simulink model "On_Board_Computer"  (R2024a)
settings: Solver=FixedStepAuto  StartTime=0.0  StopTime=10  FixedStep=sampleTime  RelTol=1e-3
values from neighbouring files (symbols this model uses):
  gains =     [workspace.mat]
settings Model: Creator=matteocolussi  LastModifiedBy=matteocolussi
settings DataIOCC: SaveOutput=off  SaveTime=off
settings ModelReferenceCC: UseModelRefSolver=on

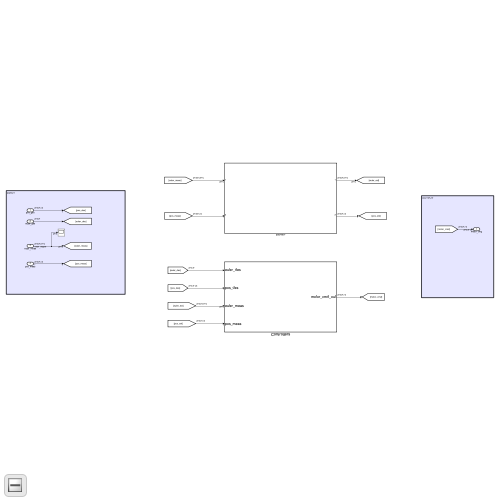
[thumbnail: Simulink's stored preview of the top-level diagram]
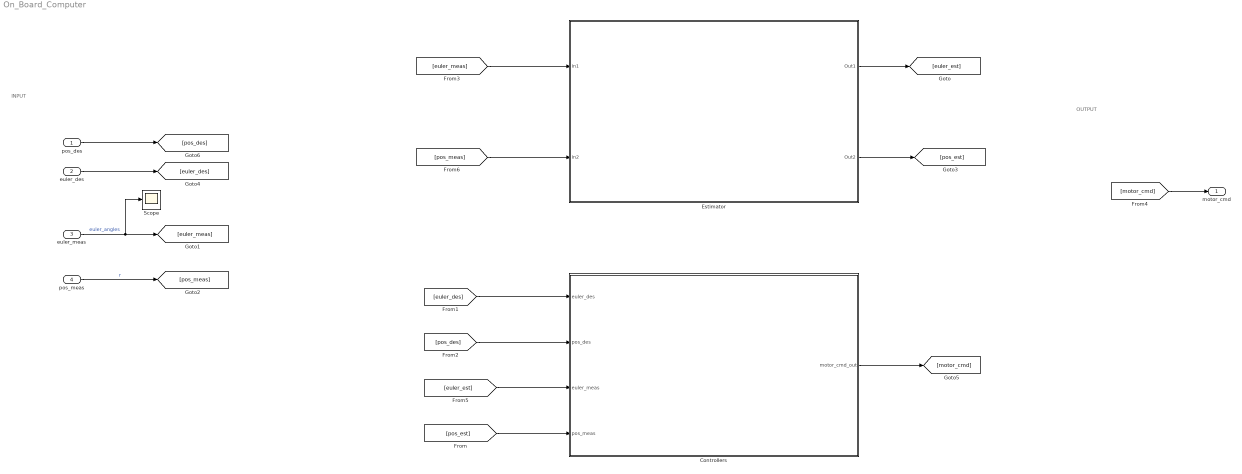
== system On_Board_Computer ==
  note: INPUT
  note: OUTPUT
  pos_des : Inport  OutDataTypeStr=double  PortDimensions=3
  euler_des : Inport  Port=2  OutDataTypeStr=double  PortDimensions=1
  euler_meas : Inport  Port=3  OutDataTypeStr=double  PortDimensions=[3 1]  SampleTime=0
  pos_meas : Inport  Port=4  OutDataTypeStr=double  PortDimensions=3  SampleTime=0
  Controllers : Subsystem
  Estimator : Subsystem
  Scope : Scope
  motor_cmd : Outport  OutDataTypeStr=double  PortDimensions=4  SampleTime=0
  wires:
  [euler_des] -> Controllers/1(euler_des)
  pos_des/1 -> [pos_des]
  pos_meas/1 -> [pos_meas]  "r"
  [pos_meas] -> Estimator/2(In2)
  [euler_meas] -> Estimator/1(In1)
  [pos_est] -> Controllers/4(pos_meas)
  euler_meas/1 -> Scope/1, [euler_meas]  "euler_angles"
  [motor_cmd] -> motor_cmd/1
  euler_des/1 -> [euler_des]
  [pos_des] -> Controllers/2(pos_des)
  Estimator/2(Out2) -> [pos_est]
  Estimator/1(Out1) -> [euler_est]
  [euler_est] -> Controllers/3(euler_meas)
  Controllers/1(motor_cmd_out) -> [motor_cmd]

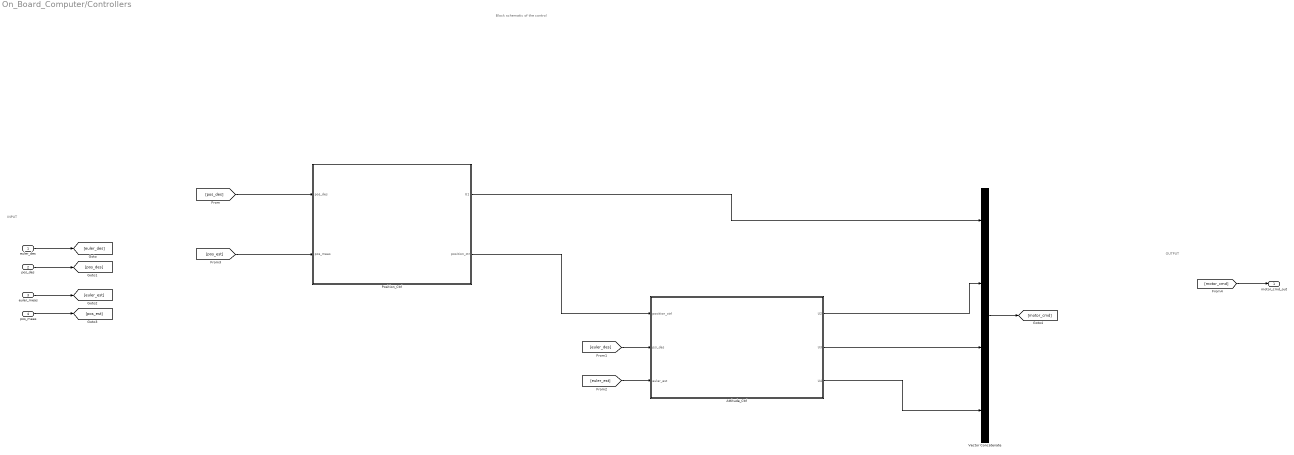
== system On_Board_Computer/Controllers ==
  note: INPUT
  note: OUTPUT
  note: Block schematic of the control
  euler_des : Inport
  pos_des : Inport  Port=2
  euler_meas : Inport  Port=3
  pos_meas : Inport  Port=4
  Attitude_Ctrl : Subsystem
  Position_Ctrl : Subsystem
  Vector Concatenate : Concatenate  NumInputs=4
  motor_cmd_out : Outport
  wires:
  [euler_des] -> Attitude_Ctrl/2(psi_des)
  Vector Concatenate/1 -> [motor_cmd]
  Attitude_Ctrl/3(U4) -> Vector Concatenate/4
  Attitude_Ctrl/2(U3) -> Vector Concatenate/3
  Attitude_Ctrl/1(U2) -> Vector Concatenate/2
  Position_Ctrl/1(U1) -> Vector Concatenate/1
  Position_Ctrl/2(position_ctrl) -> Attitude_Ctrl/1(position_ctrl)
  [pos_des] -> Position_Ctrl/1(pos_des)
  [pos_est] -> Position_Ctrl/2(pos_meas)
  [motor_cmd] -> motor_cmd_out/1
  [euler_est] -> Attitude_Ctrl/3(euler_est)
  euler_meas/1 -> [euler_est]
  pos_meas/1 -> [pos_est]
  pos_des/1 -> [pos_des]
  euler_des/1 -> [euler_des]

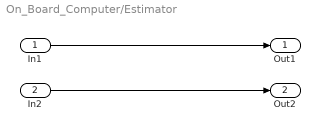
== system On_Board_Computer/Estimator ==
  In1 : Inport
  In2 : Inport  Port=2
  Out1 : Outport
  Out2 : Outport  Port=2
  wires:
  In2/1 -> Out2/1
  In1/1 -> Out1/1

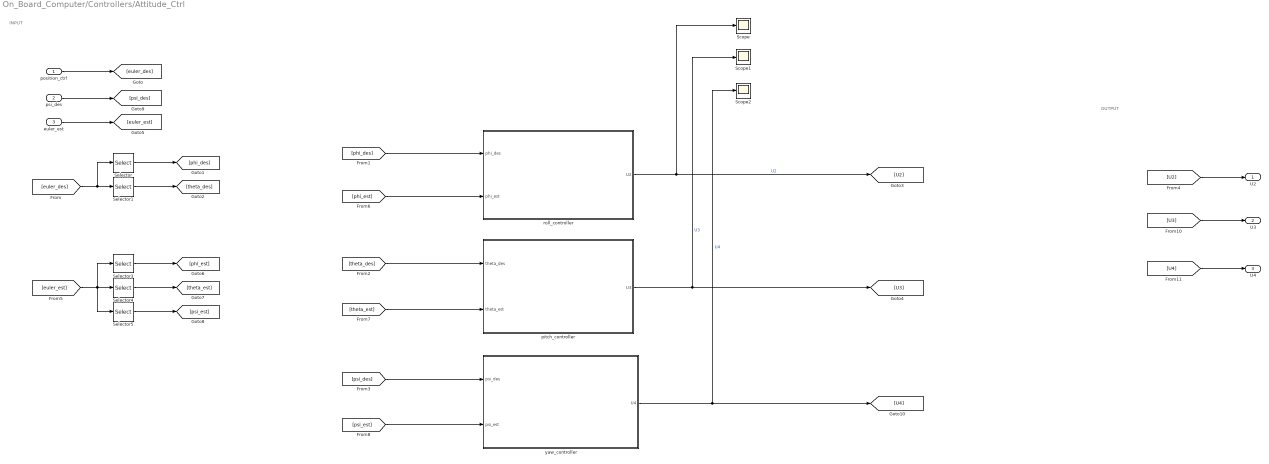
== system On_Board_Computer/Controllers/Attitude_Ctrl ==
  note: INPUT
  note: OUTPUT
  position_ctrl : Inport
  psi_des : Inport  Port=2
  euler_est : Inport  Port=3
  Scope : Scope
  Scope1 : Scope
  Scope2 : Scope
  Selector : Selector  InputPortWidth=2  IndexOptions=Index vector (dialog)  Indices=1  OutputSizes=1
  Selector1 : Selector  InputPortWidth=2  IndexOptions=Index vector (dialog)  Indices=2  OutputSizes=1
  Selector3 : Selector  InputPortWidth=3  IndexOptions=Index vector (dialog)  Indices=1  OutputSizes=1
  Selector4 : Selector  InputPortWidth=3  IndexOptions=Index vector (dialog)  Indices=2  OutputSizes=1
  Selector5 : Selector  InputPortWidth=3  IndexOptions=Index vector (dialog)  Indices=3  OutputSizes=1
  pitch_controller : Subsystem
  roll_controller : Subsystem
  yaw_controller : Subsystem
  U2 : Outport
  U3 : Outport  Port=2
  U4 : Outport  Port=3
  wires:
  psi_des/1 -> [psi_des]
  [U4] -> U4/1
  [U3] -> U3/1
  [U2] -> U2/1
  Selector3/1 -> [phi_est]
  Selector5/1 -> [psi_est]
  Selector4/1 -> [theta_est]
  [euler_est] -> Selector3/1, Selector4/1, Selector5/1
  Selector1/1 -> [theta_des]
  [euler_des] -> Selector/1, Selector1/1
  Selector/1 -> [phi_des]
  [psi_est] -> yaw_controller/2(psi_est)
  [theta_est] -> pitch_controller/2(theta_est)
  [phi_est] -> roll_controller/2(phi_est)
  euler_est/1 -> [euler_est]
  yaw_controller/1(U4) -> Scope2/1, [U4]  "U4"
  pitch_controller/1(U3) -> Scope1/1, [U3]  "U3"
  roll_controller/1(U2) -> Scope/1, [U2]  "U2"
  [psi_des] -> yaw_controller/1(psi_des)
  [theta_des] -> pitch_controller/1(theta_des)
  [phi_des] -> roll_controller/1(phi_des)
  position_ctrl/1 -> [euler_des]

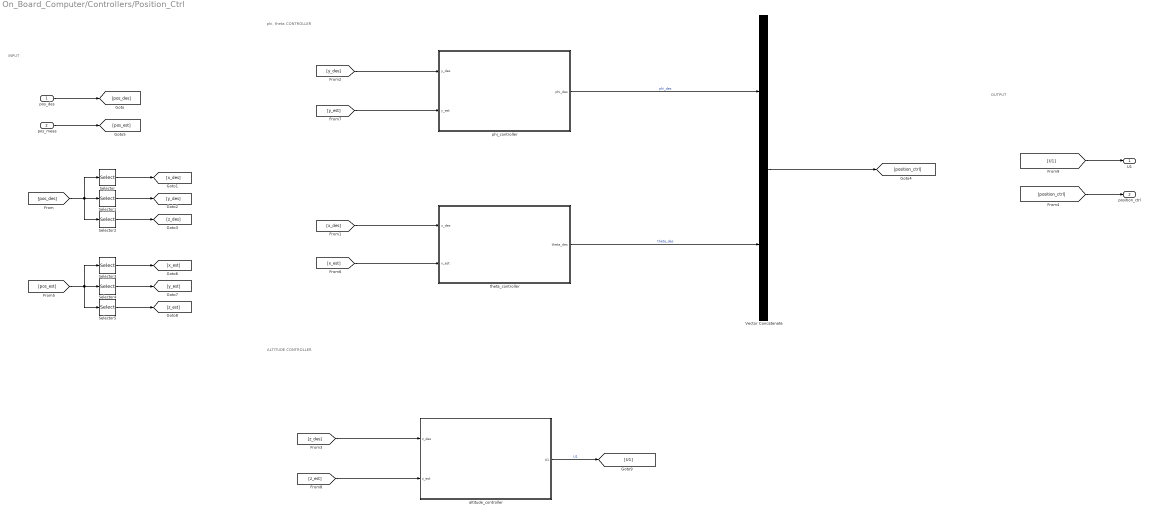
== system On_Board_Computer/Controllers/Position_Ctrl ==
  note: OUTPUT
  note: INPUT
  note: phi, theta CONTROLLER
  note: ALTITUDE CONTROLLER
  pos_des : Inport
  pos_meas : Inport  Port=2
  Selector : Selector  InputPortWidth=3  IndexOptions=Index vector (dialog)  Indices=1  OutputSizes=1
  Selector1 : Selector  InputPortWidth=3  IndexOptions=Index vector (dialog)  Indices=2  OutputSizes=1
  Selector2 : Selector  InputPortWidth=3  IndexOptions=Index vector (dialog)  Indices=3  OutputSizes=1
  Selector3 : Selector  InputPortWidth=3  IndexOptions=Index vector (dialog)  Indices=1  OutputSizes=1
  Selector4 : Selector  InputPortWidth=3  IndexOptions=Index vector (dialog)  Indices=2  OutputSizes=1
  Selector5 : Selector  InputPortWidth=3  IndexOptions=Index vector (dialog)  Indices=3  OutputSizes=1
  Vector Concatenate : Concatenate
  altitude_controller : Subsystem
  phi_controller : Subsystem
  theta_controller : Subsystem
  U1 : Outport
  position_ctrl : Outport  Port=2
  wires:
  phi_controller/1(phi_des) -> Vector Concatenate/1  "phi_des"
  [U1] -> U1/1
  altitude_controller/1(U1) -> [U1]  "U1"
  [z_des] -> altitude_controller/1(z_des)
  [z_est] -> altitude_controller/2(z_est)
  theta_controller/1(theta_des) -> Vector Concatenate/2  "theta_des"
  Vector Concatenate/1 -> [position_ctrl]
  [position_ctrl] -> position_ctrl/1
  [x_est] -> theta_controller/2(x_est)
  [y_des] -> phi_controller/1(y_des)
  [x_des] -> theta_controller/1(x_des)
  [y_est] -> phi_controller/2(y_est)
  Selector2/1 -> [z_des]
  Selector1/1 -> [y_des]
  pos_des/1 -> [pos_des]
  Selector/1 -> [x_des]
  [pos_des] -> Selector/1, Selector1/1, Selector2/1
  Selector5/1 -> [z_est]
  pos_meas/1 -> [pos_est]
  [pos_est] -> Selector3/1, Selector4/1, Selector5/1
  Selector4/1 -> [y_est]
  Selector3/1 -> [x_est]

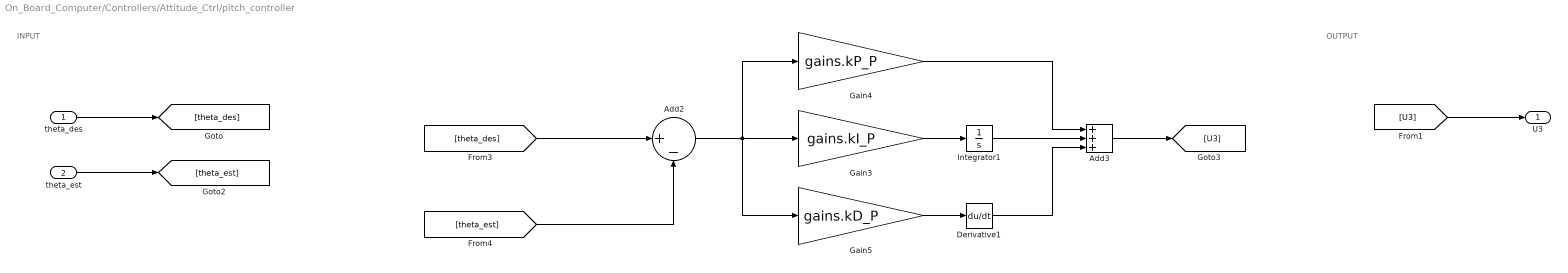
== system On_Board_Computer/Controllers/Attitude_Ctrl/pitch_controller ==
  note: INPUT
  note: OUTPUT
  theta_des : Inport
  theta_est : Inport  Port=2
  Add2 : Sum  Inputs=|+-
  Add3 : Sum  Inputs=+++
  Derivative1 : Derivative
  Gain3 : Gain  Gain=gains.kI_P
  Gain4 : Gain  Gain=gains.kP_P
  Gain5 : Gain  Gain=gains.kD_P
  Integrator1 : Integrator
  U3 : Outport
  wires:
  Gain3/1 -> Integrator1/1
  Gain5/1 -> Derivative1/1
  Add2/1 -> Gain3/1, Gain4/1, Gain5/1
  Integrator1/1 -> Add3/2
  [theta_est] -> Add2/2
  Derivative1/1 -> Add3/3
  Add3/1 -> [U3]
  Gain4/1 -> Add3/1
  [theta_des] -> Add2/1
  theta_est/1 -> [theta_est]
  theta_des/1 -> [theta_des]
  [U3] -> U3/1

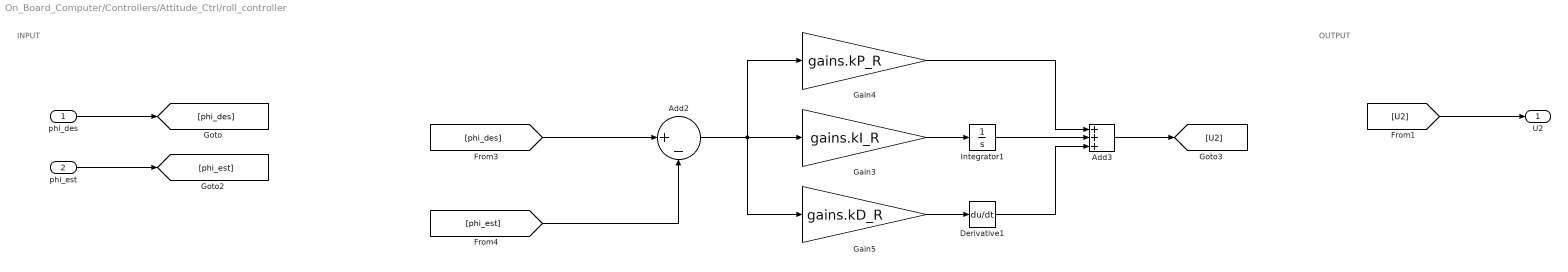
== system On_Board_Computer/Controllers/Attitude_Ctrl/roll_controller ==
  note: INPUT
  note: OUTPUT
  phi_des : Inport
  phi_est : Inport  Port=2
  Add2 : Sum  Inputs=|+-
  Add3 : Sum  Inputs=+++
  Derivative1 : Derivative
  Gain3 : Gain  Gain=gains.kI_R
  Gain4 : Gain  Gain=gains.kP_R
  Gain5 : Gain  Gain=gains.kD_R
  Integrator1 : Integrator
  U2 : Outport
  wires:
  Gain3/1 -> Integrator1/1
  Gain5/1 -> Derivative1/1
  Add2/1 -> Gain3/1, Gain4/1, Gain5/1
  Integrator1/1 -> Add3/2
  [phi_est] -> Add2/2
  Derivative1/1 -> Add3/3
  Add3/1 -> [U2]
  Gain4/1 -> Add3/1
  [phi_des] -> Add2/1
  phi_est/1 -> [phi_est]
  [U2] -> U2/1
  phi_des/1 -> [phi_des]

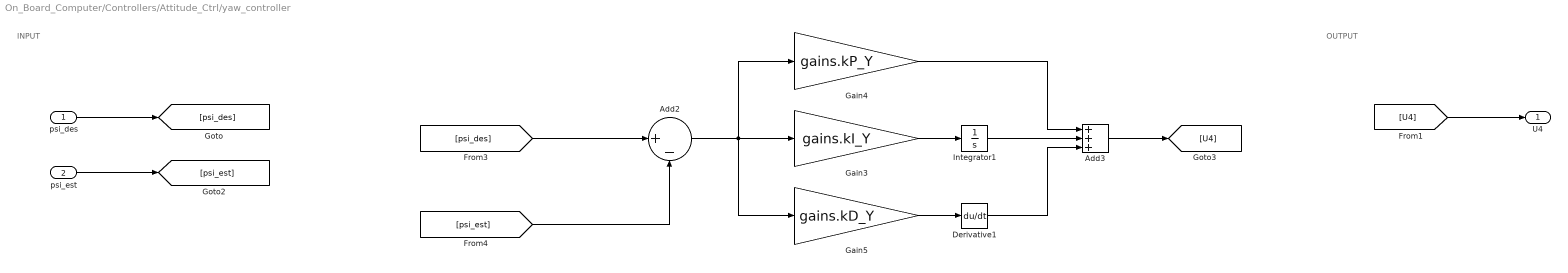
== system On_Board_Computer/Controllers/Attitude_Ctrl/yaw_controller ==
  note: INPUT
  note: OUTPUT
  psi_des : Inport
  psi_est : Inport  Port=2
  Add2 : Sum  Inputs=|+-
  Add3 : Sum  Inputs=+++
  Derivative1 : Derivative
  Gain3 : Gain  Gain=gains.kI_Y
  Gain4 : Gain  Gain=gains.kP_Y
  Gain5 : Gain  Gain=gains.kD_Y
  Integrator1 : Integrator
  U4 : Outport
  wires:
  Gain3/1 -> Integrator1/1
  Gain5/1 -> Derivative1/1
  Add2/1 -> Gain3/1, Gain4/1, Gain5/1
  Integrator1/1 -> Add3/2
  [psi_est] -> Add2/2
  Derivative1/1 -> Add3/3
  Add3/1 -> [U4]
  Gain4/1 -> Add3/1
  [psi_des] -> Add2/1
  psi_est/1 -> [psi_est]
  psi_des/1 -> [psi_des]
  [U4] -> U4/1

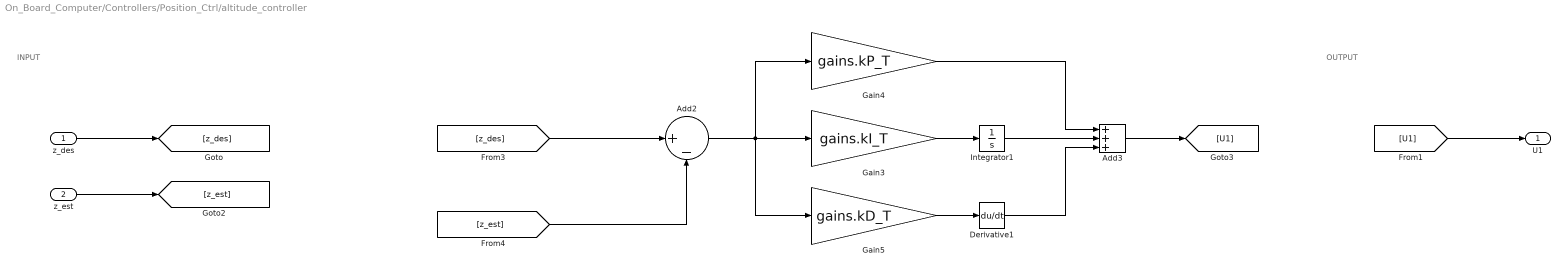
== system On_Board_Computer/Controllers/Position_Ctrl/altitude_controller ==
  note: INPUT
  note: OUTPUT
  z_des : Inport
  z_est : Inport  Port=2
  Add2 : Sum  Inputs=|+-
  Add3 : Sum  Inputs=+++
  Derivative1 : Derivative
  Gain3 : Gain  Gain=gains.kI_T
  Gain4 : Gain  Gain=gains.kP_T
  Gain5 : Gain  Gain=gains.kD_T
  Integrator1 : Integrator
  U1 : Outport
  wires:
  Gain3/1 -> Integrator1/1
  Gain5/1 -> Derivative1/1
  Add2/1 -> Gain3/1, Gain4/1, Gain5/1
  Integrator1/1 -> Add3/2
  [z_est] -> Add2/2
  Derivative1/1 -> Add3/3
  Add3/1 -> [U1]
  Gain4/1 -> Add3/1
  [z_des] -> Add2/1
  z_est/1 -> [z_est]
  z_des/1 -> [z_des]
  [U1] -> U1/1

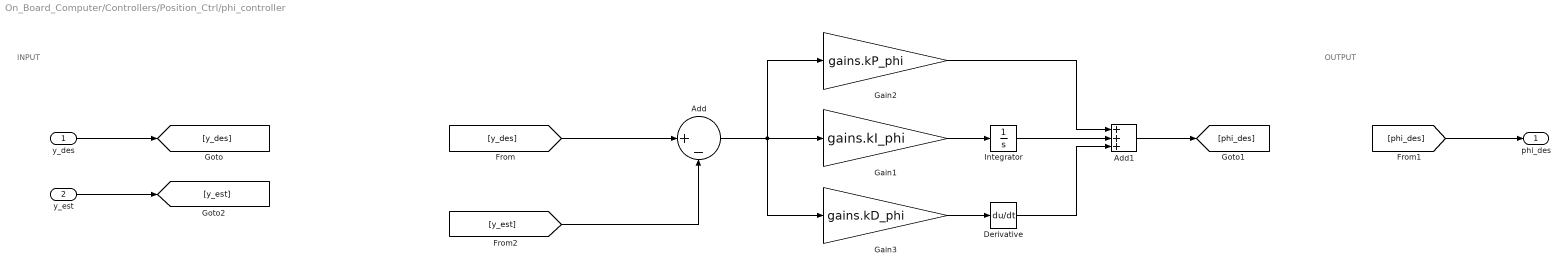
== system On_Board_Computer/Controllers/Position_Ctrl/phi_controller ==
  note: INPUT
  note: OUTPUT
  y_des : Inport
  y_est : Inport  Port=2
  Add : Sum  Inputs=|+-
  Add1 : Sum  Inputs=+++
  Derivative : Derivative
  Gain1 : Gain  Gain=gains.kI_phi
  Gain2 : Gain  Gain=gains.kP_phi
  Gain3 : Gain  Gain=gains.kD_phi
  Integrator : Integrator
  phi_des : Outport
  wires:
  Gain3/1 -> Derivative/1
  Add1/1 -> [phi_des]
  Derivative/1 -> Add1/3
  Gain2/1 -> Add1/1
  Add/1 -> Gain1/1, Gain2/1, Gain3/1
  Gain1/1 -> Integrator/1
  Integrator/1 -> Add1/2
  [y_est] -> Add/2
  y_est/1 -> [y_est]
  y_des/1 -> [y_des]
  [y_des] -> Add/1
  [phi_des] -> phi_des/1

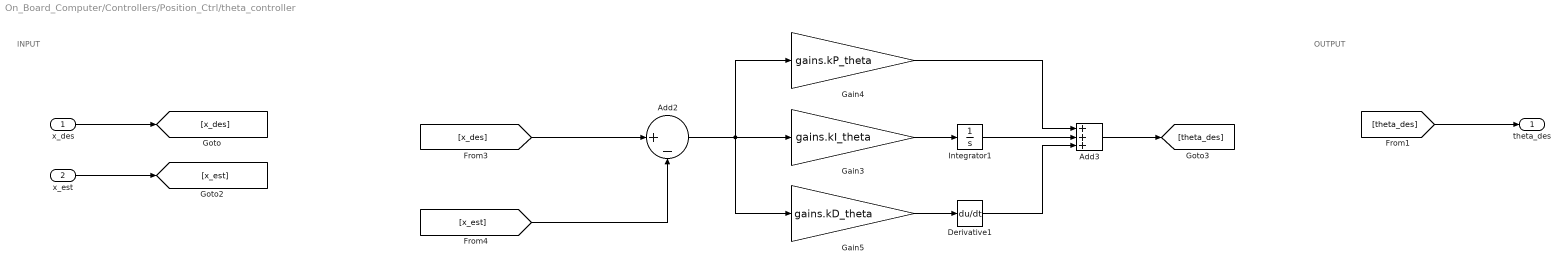
== system On_Board_Computer/Controllers/Position_Ctrl/theta_controller ==
  note: INPUT
  note: OUTPUT
  x_des : Inport
  x_est : Inport  Port=2
  Add2 : Sum  Inputs=|+-
  Add3 : Sum  Inputs=+++
  Derivative1 : Derivative
  Gain3 : Gain  Gain=gains.kI_theta
  Gain4 : Gain  Gain=gains.kP_theta
  Gain5 : Gain  Gain=gains.kD_theta
  Integrator1 : Integrator
  theta_des : Outport
  wires:
  Gain3/1 -> Integrator1/1
  Gain5/1 -> Derivative1/1
  Add2/1 -> Gain3/1, Gain4/1, Gain5/1
  Integrator1/1 -> Add3/2
  [x_est] -> Add2/2
  Derivative1/1 -> Add3/3
  Add3/1 -> [theta_des]
  Gain4/1 -> Add3/1
  [x_des] -> Add2/1
  x_est/1 -> [x_est]
  [theta_des] -> theta_des/1
  x_des/1 -> [x_des]
